simulink model "h6p12"  (R2024b)
settings: Solver=FixedStepAuto  StartTime=0.0  StopTime=25  FixedStep=.1  RelTol=1e-3
values from neighbouring files (symbols this model uses):
  noise = 1    [h6.m]
  omega_n = 2.0    (= 2)    [h6.m]
  zeta = 0.7    [h6.m]    (also in main.m)
libraries: simulink x2
settings Model: Creator=chrissheehan  LastModifiedBy=chrissheehan

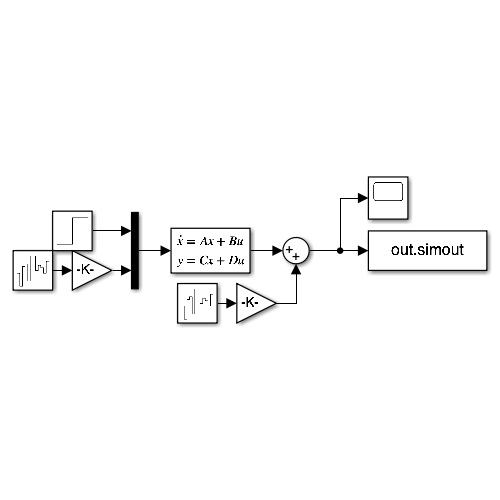
[thumbnail: Simulink's stored preview of the top-level diagram]
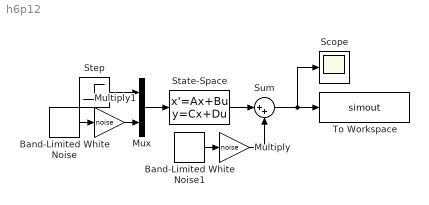
== system h6p12 ==
  Band-Limited White Noise : simulink/Sources/Band-Limited White Noise  Cov=[0.0005]  Ts=0.1  seed=[23341]
  Band-Limited White Noise1 : simulink/Sources/Band-Limited White Noise  Cov=[0.0000005]  Ts=0.1  seed=[23341]
  Multiply : Gain  Gain=noise
  Multiply1 : Gain  Gain=noise
  Mux : Mux  Inputs=2
  Scope : Scope
  State-Space : StateSpace  A=[0 1; -omega_n^2 -2*zeta*omega_n]  B=[0, 0; 1, 1]  C=[1 0]  D=[0,0]  InitialCondition=[0.05; -0.01]
  Step : Step  Time=0  SampleTime=0
  Sum : Sum  Inputs=|++
  To Workspace : ToWorkspace  VariableName=simout  SaveFormat=Timeseries  SampleTime=-1
  wires:
  State-Space/1 -> Sum/1
  Sum/1 -> To Workspace/1, Scope/1
  Mux/1 -> State-Space/1
  Step/1 -> Mux/1
  Band-Limited White Noise1/1 -> Multiply/1
  Multiply/1 -> Sum/2
  Band-Limited White Noise/1 -> Multiply1/1
  Multiply1/1 -> Mux/2
